simulink model "OCTModelLateralFlight"  (R2018b)
settings: Solver=FixedStepAuto  StartTime=0.0  StopTime=duration_s  FixedStep=0.1  MaxStep=0.1  RelTol=1e-3  AbsTol=1e-3
values from neighbouring files (symbols this model uses):
  constantNormVelBool = 0    [MMadd_ts.m]    (also in controlSurf_ts1.m; lateralFlight_ts.m)
  constantVelBool = 1    [JamesPathFollowingIntegration_ts1.m]    (also in MMadd_ts.m = 0; PathFollowingIntegration_ts1.m; controlSurf_ts1.m = 0; lateralFlight_ts.m = 0)
  constantVelMag = 7    [JamesPathFollowingIntegration_ts1.m]    (also in MMadd_ts.m = 19; PathFollowingIntegration_ts1.m = 10; controlSurf_ts1.m = 19; lateralFlight_ts.m = 34)
  env = ENV.env    [JamesPathFollowingIntegration_ts1.m]    (also in MMadd_ts.m; PathFollowingIntegration_ts1.m; controlSurf_ts1.m; controlSurf_ts2.m)
  kdRollMom = 5*MOI_X    [JamesPathFollowingIntegration_ts1.m]    (also in PathFollowingIntegration_ts1.m; lateralFlight_ts.m)
  kdVelAng = kpVelAng    (= 0.5)    [JamesPathFollowingIntegration_ts1.m]    (also in PathFollowingIntegration_ts1.m = 0.222222222222; lateralFlight_ts.m = 0.222222222222)
  kpRollMom = 2*MOI_X    [JamesPathFollowingIntegration_ts1.m]    (also in PathFollowingIntegration_ts1.m; lateralFlight_ts.m)
  kpVelAng = maxBank/(pi/2)    (= 0.5)    [JamesPathFollowingIntegration_ts1.m]    (also in PathFollowingIntegration_ts1.m = 0.222222222222; lateralFlight_ts.m = 0.222222222222)
  maxBank = 45*pi/180    (= 0.785398163397)    [JamesPathFollowingIntegration_ts1.m]    (also in PathFollowingIntegration_ts1.m = 0.349065850399; lateralFlight_ts.m = 0.349065850399)
  MMAddBool = 0    [JamesPathFollowingIntegration_ts1.m]    (also in MMadd_ts.m = 1; PathFollowingIntegration_ts1.m = 1; controlSurf_ts1.m; controlSurf_ts2.m)
  MMOverrideBool = 1    [JamesPathFollowingIntegration_ts1.m]    (also in MMadd_ts.m = 0; PathFollowingIntegration_ts1.m = 0; controlSurf_ts1.m = 0; lateralFlight_ts.m = 0)
  radialMotionBool = 0    [MMadd_ts.m]    (also in controlSurf_ts1.m; lateralFlight_ts.m)
  startControl = 15    [MMadd_ts.m]    (also in PathFollowingIntegration_ts1.m = 20; controlSurf_ts1.m; controlSurf_ts2.m = 1; controlSurf_ts3.m = 1)
  tauRollMom = .01    (= 0.01)    [JamesPathFollowingIntegration_ts1.m]    (also in PathFollowingIntegration_ts1.m; lateralFlight_ts.m)
  tauVelAng = .01    (= 0.01)    [JamesPathFollowingIntegration_ts1.m]    (also in PathFollowingIntegration_ts1.m; lateralFlight_ts.m)
  vhcl = OCT.vehicle    [JamesPathFollowingIntegration_ts1.m]    (also in MMadd_ts.m; PathFollowingIntegration_ts1.m; controlSurf_ts1.m; controlSurf_ts2.m)
undefined symbols (not defined in the file or in its folder): initAngRates, initializeVariantsFromBlock, Jinv, lateralFlightController, m, Minv, modVehicle000, modVehicle000_cl, plant, plant_cl, sim_param, sixDoFDynamics, sixDoFDynamics_ul, vehicle, vehicle_cl
libraries: vrlib x3, eulAng2RotMat_ul x3, vectorNormalizer_ul x3, setpointToOutput_cl x2, filteredPIDController_ul x2, thrAttachPtKinematics_ul x2, environment_cl x1, cartToSphere_ul x1, schmehlTangentRotation_ul x1, groundStation_cl x1, tethers_cl x1, dragTurbine_ul x1
settings Model: ExtModeTrigDuration=100  Creator=mcobb  LastModifiedBy=James Reed
settings DataIOCC: SaveOutput=off  StateSaveName=tmp_raccel_xout
settings OptimizationCC: EfficientMapNaN2IntZero=off
settings DebuggingCC: SignalRangeChecking=error
settings HardwareCC: TargetBitPerPointer=64  TargetBitPerSizeT=64  TargetBitPerPtrDiffT=64  TargetLongLongMode=on  TargetIntDivRoundTo=Zero  TargetEndianess=LittleEndian  TargetWordSize=64  TargetHWDeviceType=MATLAB Host  ProdEqTarget=off
settings RTWCC: SystemTargetFile=raccel.tlc  TemplateMakefile=raccel_default_tmf  RTWVerbose=off  RTWUseSimCustomCode=on
settings CodeAppCC: GenerateComments=off  MaxIdLength=128  MangleLength=10
settings RaccelTargetCC: GeneratePreprocessorConditionals=Use local settings  MultiInstanceERTCode=off  PreserveStateflowLocalDataDimensions=off  ENABLE_SLEXEC_SSBRIDGE=1  RTWCAPIParams=on

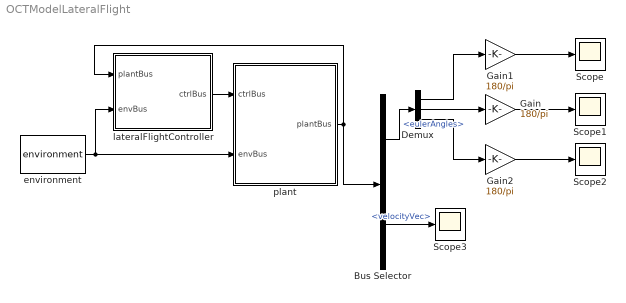
== system OCTModelLateralFlight ==
  Bus Selector : BusSelector  OutputSignals=eulerAngles,velocityVec
  Demux : Demux  Outputs=3
  Gain : Gain  Gain=180/pi
  Gain1 : Gain  Gain=180/pi
  Gain2 : Gain  Gain=180/pi
  Scope{,1..3} (4 alike) : Scope
  environment : environment_cl/environment  SystemSampleTime=-1
  lateralFlightController : Subsystem  AncestorBlock=lateralFlightController/lateralFlightController
  plant : Subsystem  AncestorBlock=plant_cl/plant  VariantControl=VSS_plant_modularPlant
  wires:
  lateralFlightController/1(ctrlBus) -> plant/1(ctrlBus)
  plant/1(plantBus) -> lateralFlightController/1(plantBus), Bus Selector/1
  environment/1 -> lateralFlightController/2(envBus), plant/2(envBus)
  Bus Selector/1 -> Demux/1  "<eulerAngles>"
  Demux/2 -> Gain/1
  Gain/1 -> Scope1/1
  Bus Selector/2 -> Scope3/1  "<velocityVec>"
  Gain2/1 -> Scope2/1
  Gain1/1 -> Scope/1
  Demux/1 -> Gain1/1
  Demux/3 -> Gain2/1

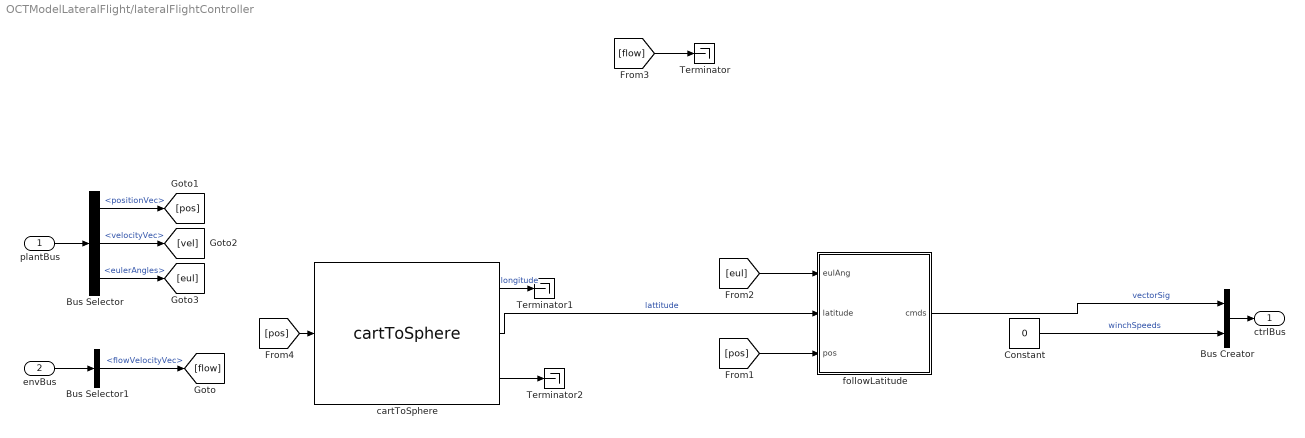
== system OCTModelLateralFlight/lateralFlightController ==
  plantBus : Inport  OutDataTypeStr=Bus: plantBus
  envBus : Inport  Port=2  OutDataTypeStr=Bus: envBus
  Bus Creator : BusCreator  Inputs=2  OutDataTypeStr=Bus: ctrlBus
  Bus Selector : BusSelector  OutputSignals=positionVec,velocityVec,eulerAngles
  Bus Selector1 : BusSelector  OutputSignals=flowVelocityVec
  Constant : Constant  Value=0
  Terminator : Terminator
  Terminator1 : Terminator
  Terminator2 : Terminator
  cartToSphere : cartToSphere_ul/cartToSphere  SystemSampleTime=-1
  followLatitude : Subsystem  mask{kpVelAngMask=kpVelAng, kdVelAngMask=kdVelAng, tauVelAngMask=tauVelAng, kpLMask=kpRollMom, kdLMask=kdRollMom, tauLMask=tauRollMom, maxBankMask=maxBank, latDes=pi/4}
      mask prompts: kpVelAngMask "Proportional Gain Velocity Angle"; kdVelAngMask "Derivative Gain Velocity Angle"; tauVelAngMask "Tau Velocity Angle"; kpLMask "Proportional Gain TanRoll"; kdLMask "Derivative Gain Tanroll"; tauLMask "Tau Roll Moment"; maxBankMask "Max Bank Angle"; latDes "Desired Latitude"
  ctrlBus : Outport  OutDataTypeStr=Bus: ctrlBus
  wires:
  [pos] -> followLatitude/3("pos ")
  cartToSphere/2 -> followLatitude/2("latitude ")  "lattitude"
  cartToSphere/3 -> Terminator2/1
  cartToSphere/1 -> Terminator1/1  "longitude"
  [pos] -> cartToSphere/1
  [flow] -> Terminator/1
  [eul] -> followLatitude/1(eulAng)
  Constant/1 -> Bus Creator/2  "winchSpeeds"
  followLatitude/1(cmds) -> Bus Creator/1  "vectorSig"
  Bus Creator/1 -> ctrlBus/1
  envBus/1 -> Bus Selector1/1
  plantBus/1 -> Bus Selector/1
  Bus Selector/2 -> [vel]  "<velocityVec>"
  Bus Selector1/1 -> [flow]  "<flowVelocityVec>"
  Bus Selector/1 -> [pos]  "<positionVec>"
  Bus Selector/3 -> [eul]  "<eulerAngles>"

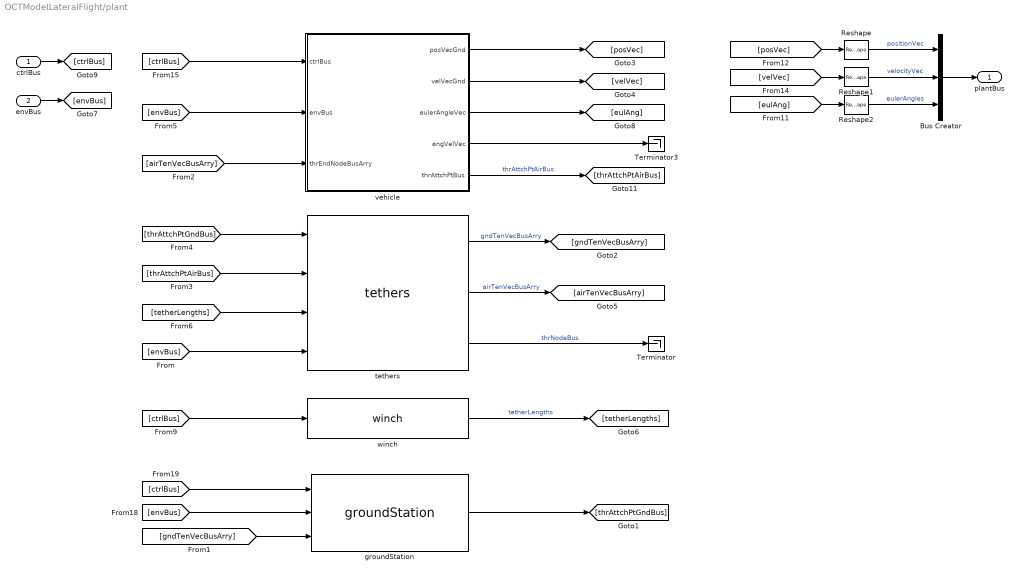
== system OCTModelLateralFlight/plant ==
  ctrlBus : Inport  OutDataTypeStr=Bus: ctrlBus
  envBus : Inport  Port=2  OutDataTypeStr=Bus: envBus
  Bus Creator : BusCreator  Inputs=3  OutDataTypeStr=Bus: plantBus
  Reshape : Reshape  OutputDimensionality=Column vector (2-D)
  Reshape1 : Reshape  OutputDimensionality=Column vector (2-D)
  Reshape2 : Reshape  OutputDimensionality=Column vector (2-D)
  Terminator : Terminator
  Terminator3 : Terminator
  groundStation : groundStation_cl/groundStation  SystemSampleTime=-1
  tethers : tethers_cl/tethers  SystemSampleTime=-1
      link override tether000: numNodes=thr.tether1.numNodes.Value
  vehicle : Subsystem  AncestorBlock=vehicle_cl/vehicle  LoadFcn=initializeVariantsFromBlock(gcb)  InitFcn=initializeVariantsFromBlock(gcb)  StartFcn=initializeVariantsFromBlock(gcb)  Variant=on
      settings: PreSaveFcn=initializeVariantsFromBlock(gcb)
  winch : winch_cl/winch  SystemSampleTime=-1
  plantBus : Outport  OutDataTypeStr=Bus: plantBus
  wires:
  [ctrlBus] -> winch/1
  [envBus] -> vehicle/2(envBus)
  [ctrlBus] -> vehicle/1(ctrlBus)
  [ctrlBus] -> groundStation/1
  [envBus] -> groundStation/2
  [tetherLengths] -> tethers/3
  [thrAttchPtGndBus] -> tethers/1
  [thrAttchPtAirBus] -> tethers/2
  [airTenVecBusArry] -> vehicle/3(thrEndNodeBusArry)
  [gndTenVecBusArry] -> groundStation/3
  tethers/3 -> Terminator/1  "thrNodeBus"
  tethers/2 -> [airTenVecBusArry]  "airTenVecBusArry"
  tethers/1 -> [gndTenVecBusArry]  "gndTenVecBusArry"
  groundStation/1 -> [thrAttchPtGndBus]
  [envBus] -> tethers/4
  vehicle/4(angVelVec) -> Terminator3/1
  vehicle/2(velVecGnd) -> [velVec]
  vehicle/5(thrAttchPtBus) -> [thrAttchPtAirBus]  "thrAttchPtAirBus"
  vehicle/1(posVecGnd) -> [posVec]
  vehicle/3(eulerAngleVec) -> [eulAng]
  [eulAng] -> Reshape2/1
  [velVec] -> Reshape1/1
  [posVec] -> Reshape/1
  winch/1 -> [tetherLengths]  "tetherLengths"
  Reshape1/1 -> Bus Creator/2  "velocityVec"
  Reshape2/1 -> Bus Creator/3  "eulerAngles"
  Reshape/1 -> Bus Creator/1  "positionVec"
  Bus Creator/1 -> plantBus/1
  ctrlBus/1 -> [ctrlBus]
  envBus/1 -> [envBus]

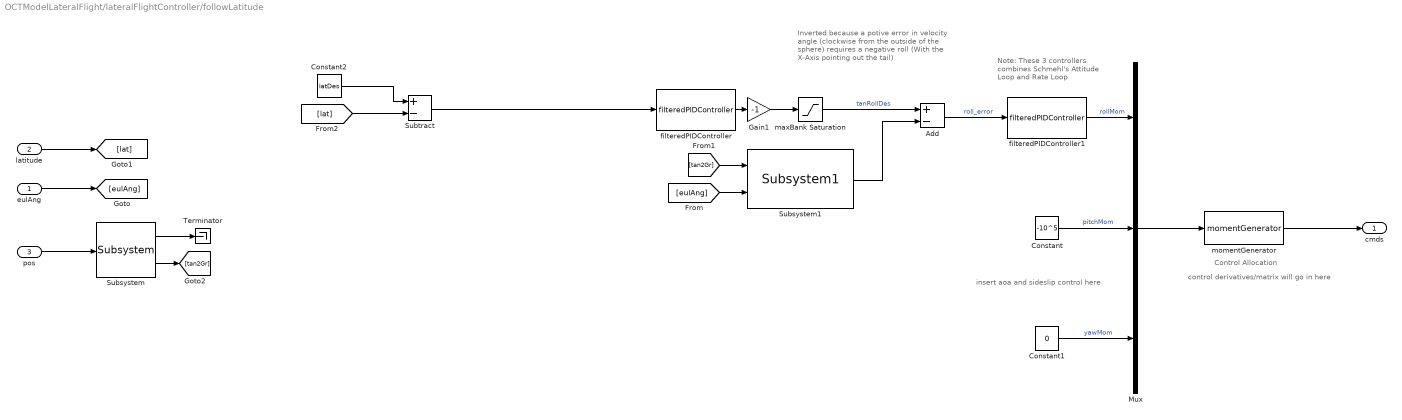
== system OCTModelLateralFlight/lateralFlightController/followLatitude ==
  note: Note: These 3 controllers
      | combines Schmehl's Attitude
      | Loop and Rate Loop
  note: Inverted because a potive error
      | in velocity angle (clockwise from the
      | outside of the sphere) requires a negative
      | roll (With the X-Axis pointing out the tail)
  note: Control Allocation
  note: insert aoa and sideslip control here
  note: control derivatives/matrix will go in here
  eulAng : Inport
  "latitude " : Inport  Port=2
  "pos " : Inport  Port=3
  Add : Sum  Inputs=+-
  Constant : Constant  Value=-10^5
  Constant1 : Constant  Value=0
  Constant2 : Constant  Value=latDes
  Gain1 : Gain  Gain=-1
  Mux : Mux  Inputs=3
  Subsystem : schmehlTangentRotation_ul/Subsystem  SystemSampleTime=-1
  Subsystem1 : setpointToOutput_cl/Subsystem/Subsystem1  SystemSampleTime=-1
  Subtract : Sum  Inputs=+-
  Terminator : Terminator
  filteredPIDController : filteredPIDController_ul/filteredPIDController  kp=kpVelAngMask  ki=0  kd=kdVelAngMask  Value=tauVelAngMask
  filteredPIDController1 : filteredPIDController_ul/filteredPIDController  kp=kpLMask  ki=0  kd=kdLMask  Value=tauLMask
  maxBank Saturation : Saturate  UpperLimit=maxBankMask  LowerLimit=-maxBankMask
  momentGenerator : setpointToOutput_cl/Subsystem/momentGenerator  SystemSampleTime=-1
  cmds : Outport
  wires:
  Subsystem/1 -> Terminator/1
  Subsystem/2 -> [tan2Gr]
  "pos "/1 -> Subsystem/1
  Subtract/1 -> filteredPIDController/1
  Constant2/1 -> Subtract/1
  [lat] -> Subtract/2
  "latitude "/1 -> [lat]
  momentGenerator/1 -> cmds/1
  Mux/1 -> momentGenerator/1
  maxBank Saturation/1 -> Add/1  "tanRollDes"
  Constant/1 -> Mux/2  "pitchMom"
  [eulAng] -> Subsystem1/2
  filteredPIDController1/1 -> Mux/1  "rollMom"
  filteredPIDController/1 -> Gain1/1
  eulAng/1 -> [eulAng]
  Subsystem1/1 -> Add/2
  Gain1/1 -> maxBank Saturation/1
  Add/1 -> filteredPIDController1/1  "roll_error"
  Constant1/1 -> Mux/3  "yawMom"
  [tan2Gr] -> Subsystem1/1

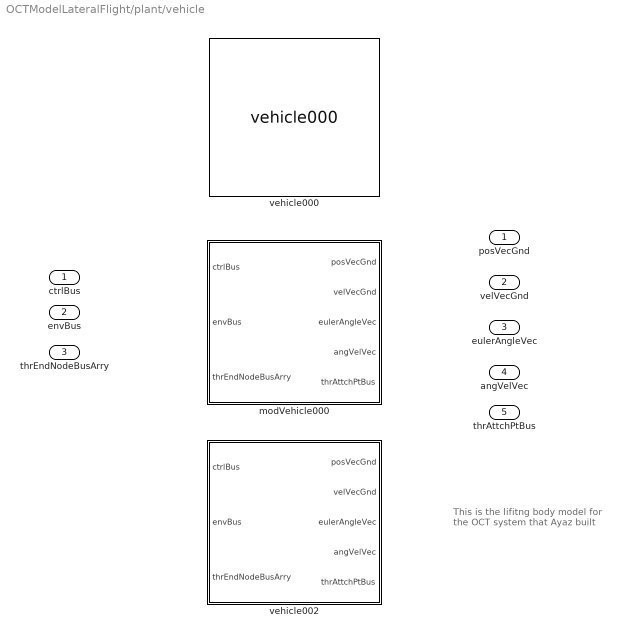
== system OCTModelLateralFlight/plant/vehicle ==
  note: This is the lifitng body model for the OCT system that Ayaz built
  ctrlBus : Inport  OutDataTypeStr=Bus: ctrlBus
  envBus : Inport  Port=2  OutDataTypeStr=Bus: envBus
  thrEndNodeBusArry : Inport  Port=3
  modVehicle000 : Subsystem  AncestorBlock=modVehicle000_cl/modVehicle000  VariantControl=VSS_vehicle_modVehicle000  mask{vcl=vhcl, rho=env.water.density.Value, grav=env.gravAccel.Value}
      mask prompts: vcl "Vehicle"; rho "Fluid Density"; grav "Gravity"
      mask DialogControl Container9 Prompt: General
      mask DialogControl Container5 Prompt: Vehicle object
      mask DialogControl ParameterGroupVar Prompt: Environmental
      mask Display:
      | image('kite.jpg',[100 100 601 528]/4,'on')
      | 
      | port_label('input',1,'ctrlBus')
      | port_label('input',2,'envBus')
      | port_label('input',3,'thrEndNodeBusArry')
      | 
      | port_label('output',1,'posVecGnd')
      | port_label('output',2,'velVecGnd')
      | port_label('output',3,'eulAng')
      | port_label('output',4,'angVelVec')
      | port_label('output',5,'thrAttchPtBus')
  vehicle000 : vehicle000_cl/vehicle000  VariantControl=VSS_vehicle_vehicle000  vcl=vhcl  rho=env.water.density.Value  grav=env.gravAccel.Value
  vehicle002 : Subsystem  VariantControl=VSS_vehicle_vehicle002
      mask init:
      | load('OrginalOCctModelVars');
  posVecGnd : Outport
  velVecGnd : Outport  Port=2
  eulerAngleVec : Outport  Port=3
  angVelVec : Outport  Port=4
  thrAttchPtBus : Outport  Port=5

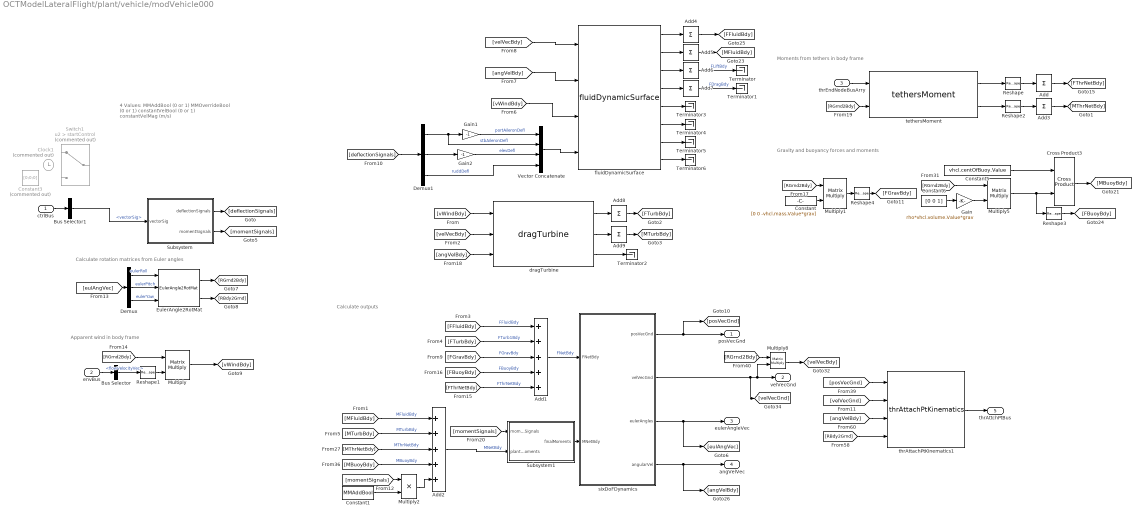
== system OCTModelLateralFlight/plant/vehicle/modVehicle000 ==
  note: Moments from tethers in body frame
  note: Gravity and buoyancy forces and moments
  note: Calculate rotation matrices from Euler angles
  note: Apparent wind in body frame
  note: Calculate outputs
  note: 4 Values:
      | MMAddBool (0 or 1)
      | MMOverrideBool (0 or 1)
      | constantVelBool (0 or 1)
      | constantVelMag (m/s)
  ctrlBus : Inport  OutDataTypeStr=Bus: ctrlBus
  envBus : Inport  Port=2  OutDataTypeStr=Bus: envBus
  thrEndNodeBusArry : Inport  Port=3
  Add : Sum  Inputs=+  CollapseMode=Specified dimension  CollapseDim=2
  Add1 : Sum  Inputs=+++++
  Add2 : Sum  Inputs=+++++
  Add3 : Sum  Inputs=+  CollapseMode=Specified dimension  CollapseDim=2
  Add{4..9} (6 alike) : Sum  Inputs=1  CollapseMode=Specified dimension  CollapseDim=2
  Bus Selector : BusSelector  OutputSignals=flowVelocityVec
  Bus Selector1 : BusSelector  OutputSignals=vectorSig
  Clock1 : Clock  Commented=on
  Constant : Constant  Value=[0 0 -vhcl.mass.Value*grav]
  Constant1 : Constant  Value=MMAddBool
  Constant3 : Constant  Commented=on  Value=[0;0;0]
  Constant5 : Constant  Value=vhcl.centOfBuoy.Value
  Constant6 : Constant  Value=[0 0 1]
  Cross Product3 : vrlib/Utilities/Cross Product
      settings: SourceProductBaseCode=VR
  Demux : Demux  Outputs=3
  Demux1 : Demux  Outputs=3
  EulerAngle2RotMat : eulAng2RotMat_ul/EulerAngle2RotMat  SystemSampleTime=-1
  Gain : Gain  Gain=rho*vhcl.volume.Value*grav
  Gain1 : Gain  Gain=-1
  Gain2 : Gain  Gain=-1
  Multiply{,1,5,8} (4 alike) : Product  Multiplication=Matrix(*)
  Multiply2 : Product
  Reshape : Reshape  OutputDimensionality=Customize  OutputDimensions=[3 vhcl.numTethers.Value]
  Reshape1 : Reshape  OutputDimensionality=Column vector (2-D)
  Reshape2 : Reshape  OutputDimensionality=Customize  OutputDimensions=[3 vhcl.numTethers.Value]
  Reshape3 : Reshape  OutputDimensionality=Column vector (2-D)
  Reshape4 : Reshape  OutputDimensionality=Column vector (2-D)
  Subsystem : Subsystem
  Subsystem1 : Subsystem
  Switch1 : Switch  Commented=on  Criteria=u2 > Threshold  Threshold=startControl
  Terminator{,1..6} (7 alike) : Terminator
  Vector Concatenate : Concatenate  NumInputs=4
  dragTurbine : dragTurbine_ul/dragTurbine  rho_fluid=rho  turb_struct=vhcl.struct('OCT.turb')
  fluidDynamicSurface : fluidDynamicSurface_cl/fluidDynamicSurface  aeroStruct=vcl.struct('OCT.aeroSurf')  fluidDensity=rho
  sixDoFDynamics : Subsystem  AncestorBlock=sixDoFDynamics_ul/sixDoFDynamics  mask{M=vhcl.mass.Value, J=vhcl.inertia.Value, initPos=vhcl.initPosVecGnd.Value, initVel=vhcl.initVelVecGnd.Value, initEulAngs=vhcl.initEulAngBdy.Value, initAngVel=vhcl.initAngVelVecBdy.Value}
      mask prompts: M "Mass"; J "Inertia matrix"; initPos "Initial position"; initVel "Initial velocity"; initEulAngs "Initial Euler Angles"; initAngVel "Initial Angular Velocity Vec"
      mask init:
      | sixDoFDynamics_init
  tethersMoment : tethersMoment_cl/tethersMoment  arms=vhcl.struct('OCT.thrAttch')
  thrAttachPtKinematics1 : thrAttachPtKinematics_ul/thrAttachPtKinematics  atchPts=vhcl.struct('OCT.thrAttch')
  posVecGnd : Outport
  velVecGnd : Outport  Port=2
  eulerAngleVec : Outport  Port=3
  angVelVec : Outport  Port=4
  thrAttchPtBus : Outport  Port=5
  wires:
  Bus Selector1/1 -> Subsystem/1(vectorSig)  "<vectorSig>"
  fluidDynamicSurface/8 -> Terminator6/1
  Subsystem/2(momentSignals) -> [momentSignals]
  Reshape4/1 -> [FGravBdy]
  Multiply1/1 -> Reshape4/1
  Reshape3/1 -> [FBuoyBdy]
  fluidDynamicSurface/6 -> Terminator4/1
  fluidDynamicSurface/7 -> Terminator5/1
  fluidDynamicSurface/5 -> Terminator3/1
  Constant1/1 -> Multiply2/2
  Multiply2/1 -> Add2/5
  [momentSignals] -> Multiply2/1
  sixDoFDynamics/2(velVecGnd) -> [velVecGnd], Multiply8/2, velVecGnd/1
  [momentSignals] -> Subsystem1/1(momentSignals)
  Add2/1 -> Subsystem1/2("plantCreatedMoments ")  "MNetBdy"
  Subsystem1/1(finalMoments) -> sixDoFDynamics/2(MNetBdy)
  Subsystem/1(deflectionSignals) -> [deflectionSignals]
  Gain2/1 -> Vector Concatenate/3  "elevDefl"
  Demux1/1 -> Gain1/1, Vector Concatenate/2  "stbAileronDefl"
  Gain1/1 -> Vector Concatenate/1  "portAileronDefl"
  Demux1/2 -> Gain2/1
  Demux1/3 -> Vector Concatenate/4  "ruddDefl"
  [deflectionSignals] -> Demux1/1
  ctrlBus/1 -> Bus Selector1/1
  Vector Concatenate/1 -> fluidDynamicSurface/4
  Gain/1 -> Multiply5/2
  [FGravBdy] -> Add1/3  "FGravBdy"
  [FBuoyBdy] -> Add1/4  "FBuoyBdy"
  [FThrNetBdy] -> Add1/5  "FThrNetBdy"
  [MBuoyBdy] -> Add2/4  "MBuoyBdy"
  [angVelBdy] -> dragTurbine/3
  [velVecBdy] -> dragTurbine/2
  [vWindBdy] -> dragTurbine/1
  dragTurbine/3 -> Terminator2/1
  Add9/1 -> [MTurbBdy]
  Add8/1 -> [FTurbBdy]
  dragTurbine/2 -> Add9/1
  dragTurbine/1 -> Add8/1
  Add7/1 -> Terminator1/1  "FDragBdy"
  Add6/1 -> Terminator/1  "FLiftBdy"
  Add5/1 -> [MFluidBdy]
  Add4/1 -> [FFluidBdy]
  [velVecBdy] -> fluidDynamicSurface/1
  [angVelBdy] -> fluidDynamicSurface/2
  [vWindBdy] -> fluidDynamicSurface/3
  fluidDynamicSurface/4 -> Add7/1
  fluidDynamicSurface/3 -> Add6/1
  fluidDynamicSurface/1 -> Add4/1
  envBus/1 -> Bus Selector/1
  Add1/1 -> sixDoFDynamics/1(FNetBdy)  "FNetBdy"
  tethersMoment/2 -> Reshape2/1
  Reshape2/1 -> Add3/1
  Add3/1 -> [MThrNetBdy]
  Reshape1/1 -> Multiply/2
  [RGrnd2Bdy] -> tethersMoment/2
  Add/1 -> [FThrNetBdy]
  Reshape/1 -> Add/1
  tethersMoment/1 -> Reshape/1
  [velVecGnd] -> thrAttachPtKinematics1/2
  [RBdy2Grnd] -> thrAttachPtKinematics1/4
  [posVecGnd] -> thrAttachPtKinematics1/1
  thrAttachPtKinematics1/1 -> thrAttchPtBus/1
  [angVelBdy] -> thrAttachPtKinematics1/3
  [RGrnd2Bdy] -> Multiply8/1
  Multiply8/1 -> [velVecBdy]
  sixDoFDynamics/1(posVecGnd) -> posVecGnd/1, [posVecGnd]
  fluidDynamicSurface/2 -> Add5/1
  Constant/1 -> Multiply1/2
  [FTurbBdy] -> Add1/2  "FTurb1Bdy"
  [FFluidBdy] -> Add1/1  "FFluidBdy"
  sixDoFDynamics/4(angularVel) -> angVelVec/1, [angVelBdy]
  sixDoFDynamics/3(eulerAngles) -> eulerAngleVec/1, [eulAngVec]
  [MTurbBdy] -> Add2/2  "MTurbBdy"
  [MThrNetBdy] -> Add2/3  "MThrNetBdy"
  [MFluidBdy] -> Add2/1  "MFluidBdy"
  Constant5/1 -> Cross Product3/1
  Cross Product3/1 -> [MBuoyBdy]
  [RGrnd2Bdy] -> Multiply5/1
  Multiply5/1 -> Reshape3/1, Cross Product3/2
  Constant6/1 -> Gain/1
  thrEndNodeBusArry/1 -> tethersMoment/1
  [RGrnd2Bdy] -> Multiply1/1
  Multiply/1 -> [vWindBdy]
  [RGrnd2Bdy] -> Multiply/1
  EulerAngle2RotMat/2 -> [RBdy2Grnd]
  EulerAngle2RotMat/1 -> [RGrnd2Bdy]
  Demux/3 -> EulerAngle2RotMat/3  "eulerYaw"
  Demux/1 -> EulerAngle2RotMat/1  "eulerRoll"
  Demux/2 -> EulerAngle2RotMat/2  "eulerPitch"
  [eulAngVec] -> Demux/1
  Bus Selector/1 -> Reshape1/1  "<flowVelocityVec>"

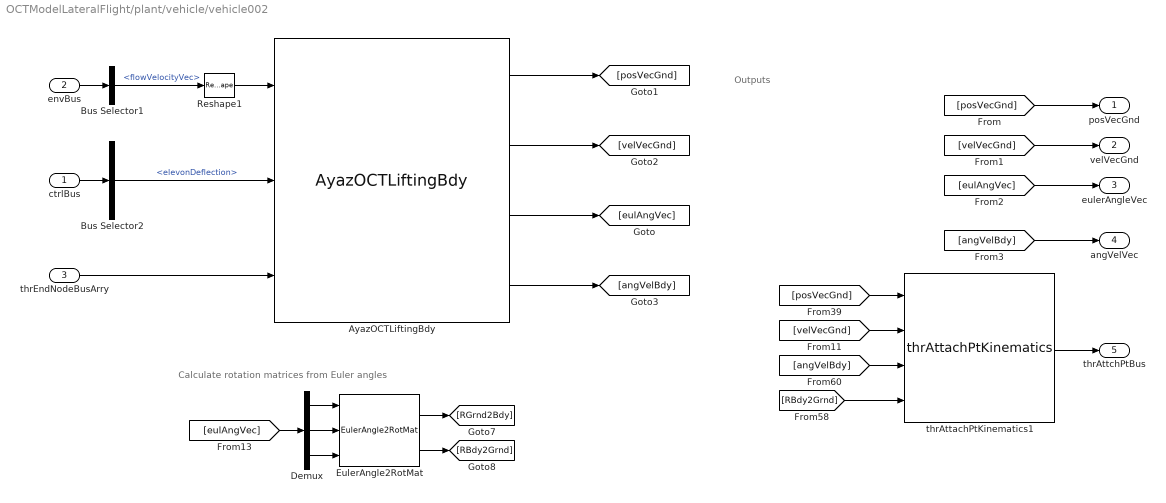
== system OCTModelLateralFlight/plant/vehicle/vehicle002 ==
  note: Calculate rotation matrices from Euler angles
  note: Outputs
  ctrlBus : Inport  OutDataTypeStr=Bus: ctrlBus
  envBus : Inport  Port=2  OutDataTypeStr=Bus: envBus
  thrEndNodeBusArry : Inport  Port=3
  AyazOCTLiftingBdy : AyazOctLiftingBdy_cl/AyazOCTLiftingBdy  sim_param=sim_param  initCon=origOCT_iniCon
  Bus Selector1 : BusSelector  OutputSignals=flowVelocityVec
  Bus Selector2 : BusSelector  OutputSignals=elevonDeflection
  Demux : Demux  Outputs=3
  EulerAngle2RotMat : eulAng2RotMat_ul/EulerAngle2RotMat  SystemSampleTime=-1
  Reshape1 : Reshape  OutputDimensionality=Column vector (2-D)
  thrAttachPtKinematics1 : thrAttachPtKinematics_ul/thrAttachPtKinematics  atchPts=[sim_param.tether_imp_nodes.R1n_cm,sim_param.tether_imp_nodes.R2n_cm,sim_param.tether_imp_nodes.R3n_cm]
  posVecGnd : Outport
  velVecGnd : Outport  Port=2
  eulerAngleVec : Outport  Port=3
  angVelVec : Outport  Port=4
  thrAttchPtBus : Outport  Port=5
  wires:
  [angVelBdy] -> angVelVec/1
  [eulAngVec] -> eulerAngleVec/1
  [velVecGnd] -> velVecGnd/1
  [posVecGnd] -> posVecGnd/1
  AyazOCTLiftingBdy/4 -> [angVelBdy]
  AyazOCTLiftingBdy/2 -> [velVecGnd]
  AyazOCTLiftingBdy/1 -> [posVecGnd]
  AyazOCTLiftingBdy/3 -> [eulAngVec]
  EulerAngle2RotMat/2 -> [RBdy2Grnd]
  EulerAngle2RotMat/1 -> [RGrnd2Bdy]
  Demux/1 -> EulerAngle2RotMat/1
  Demux/2 -> EulerAngle2RotMat/2
  [eulAngVec] -> Demux/1
  Demux/3 -> EulerAngle2RotMat/3
  [velVecGnd] -> thrAttachPtKinematics1/2
  [angVelBdy] -> thrAttachPtKinematics1/3
  thrAttachPtKinematics1/1 -> thrAttchPtBus/1
  [RBdy2Grnd] -> thrAttachPtKinematics1/4
  [posVecGnd] -> thrAttachPtKinematics1/1
  thrEndNodeBusArry/1 -> AyazOCTLiftingBdy/3
  Bus Selector2/1 -> AyazOCTLiftingBdy/2  "<elevonDeflection>"
  ctrlBus/1 -> Bus Selector2/1
  envBus/1 -> Bus Selector1/1
  Reshape1/1 -> AyazOCTLiftingBdy/1
  Bus Selector1/1 -> Reshape1/1  "<flowVelocityVec>"

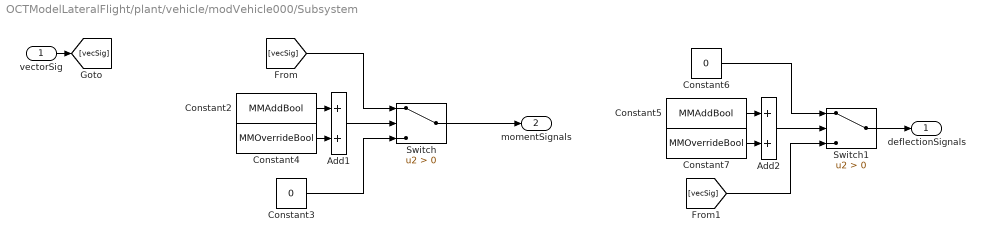
== system OCTModelLateralFlight/plant/vehicle/modVehicle000/Subsystem ==
  vectorSig : Inport
  Add1 : Sum
  Add2 : Sum
  Constant2 : Constant  Value=MMAddBool
  Constant3 : Constant  Value=0
  Constant4 : Constant  Value=MMOverrideBool
  Constant5 : Constant  Value=MMAddBool
  Constant6 : Constant  Value=0
  Constant7 : Constant  Value=MMOverrideBool
  Switch : Switch  Criteria=u2 > Threshold
  Switch1 : Switch  Criteria=u2 > Threshold
  deflectionSignals : Outport
  momentSignals : Outport  Port=2
  wires:
  Constant6/1 -> Switch1/1
  vectorSig/1 -> [vecSig]
  Switch1/1 -> deflectionSignals/1
  Add2/1 -> Switch1/2
  Constant5/1 -> Add2/1
  Constant7/1 -> Add2/2
  [vecSig] -> Switch1/3
  Switch/1 -> momentSignals/1
  Constant4/1 -> Add1/2
  Constant2/1 -> Add1/1
  Add1/1 -> Switch/2
  [vecSig] -> Switch/1
  Constant3/1 -> Switch/3

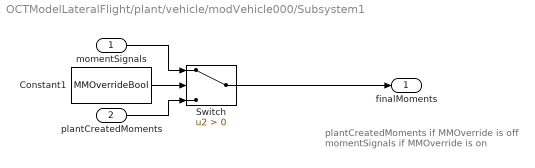
== system OCTModelLateralFlight/plant/vehicle/modVehicle000/Subsystem1 ==
  note: plantCreatedMoments if MMOverride is off
      | momentSignals if MMOverride is on
  momentSignals : Inport
  "plantCreatedMoments " : Inport  Port=2
  Constant1 : Constant  Value=MMOverrideBool
  Switch : Switch  Criteria=u2 > Threshold
  finalMoments : Outport
  wires:
  Switch/1 -> finalMoments/1
  "plantCreatedMoments "/1 -> Switch/3
  momentSignals/1 -> Switch/1
  Constant1/1 -> Switch/2

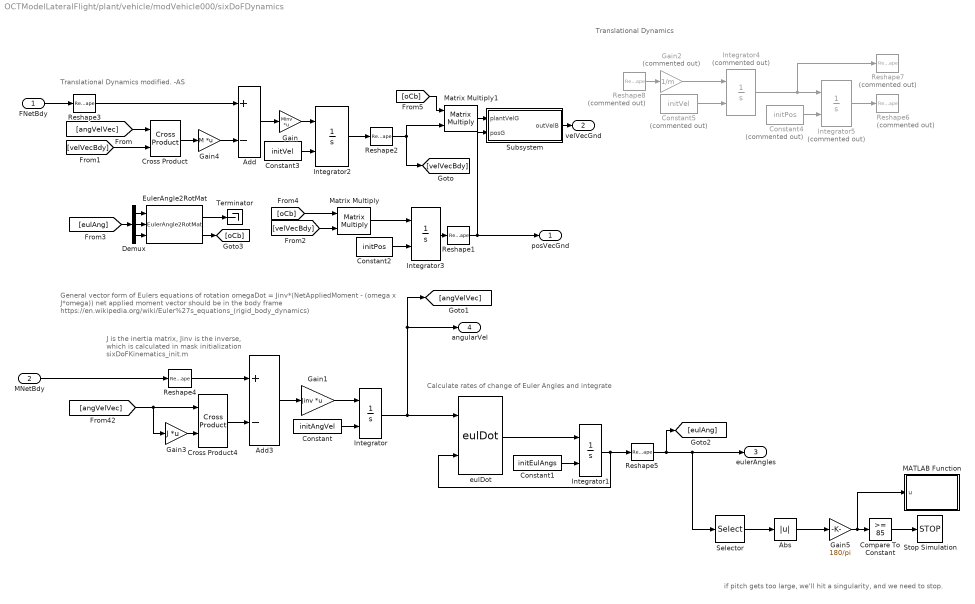
== system OCTModelLateralFlight/plant/vehicle/modVehicle000/sixDoFDynamics ==
  note: if pitch gets too large, we'll hit a singularity, and we need to stop.
  note: Translational Dynamics modified. -AS
  note: Calculate rates of change of Euler Angles and integrate
  note: General vector form of Eulers equations of rotation
      | omegaDot = Jinv*(NetAppliedMoment - (omega x J*omega))
      | net applied moment vector should be in the body frame
      | https://en.wikipedia.org/wiki/Euler%27s_equations_(rigid_body_dynamics)
  note: J is the inertia matrix, Jinv is the inverse,
      | which is calculated in mask initialization
      | sixDoFKinematics_init.m
  note: Translational Dynamics
  FNetBdy : Inport
  MNetBdy : Inport  Port=2
  Abs : Abs
  Add : Sum  Inputs=+-
  Add3 : Sum  Inputs=+-
  Compare To Constant : simulink/Logic and Bit Operations/Compare To Constant  relop=>=  const=85  OutDataTypeStr=boolean
  Constant : Constant  Value=initAngVel
  Constant1 : Constant  Value=initEulAngs
  Constant2 : Constant  Value=initPos
  Constant3 : Constant  Value=initVel
  Constant4 : Constant  Commented=on  Value=initPos
  Constant5 : Constant  Commented=on  Value=initVel
  Cross Product : vrlib/Utilities/Cross Product
      settings: SourceProductBaseCode=VR
  Cross Product4 : vrlib/Utilities/Cross Product
      settings: SourceProductBaseCode=VR
  Demux : Demux  Outputs=3
  EulerAngle2RotMat : eulAng2RotMat_ul/EulerAngle2RotMat  SystemSampleTime=-1
  Gain : Gain  Gain=Minv  Multiplication=Matrix(K*u)
  Gain1 : Gain  Gain=Jinv  Multiplication=Matrix(K*u)
  Gain2 : Gain  Commented=on  Gain=1/m
  Gain3 : Gain  Gain=J  Multiplication=Matrix(K*u)
  Gain4 : Gain  Gain=M  Multiplication=Matrix(K*u)
  Gain5 : Gain  Gain=180/pi
  Integrator : Integrator  InitialConditionSource=external  InitialCondition=initAngRates
  Integrator1 : Integrator  InitialConditionSource=external  InitialCondition=initEulAngs
  Integrator2 : Integrator  InitialConditionSource=external  InitialCondition=initVel
  Integrator3 : Integrator  InitialConditionSource=external  InitialCondition=initPos
  Integrator4 : Integrator  Commented=on  InitialConditionSource=external  InitialCondition=initVel
  Integrator5 : Integrator  Commented=on  InitialConditionSource=external  InitialCondition=initPos
  MATLAB Function : MATLAB Function  TreatAsAtomicUnit=on
  Matrix Multiply : Product  Multiplication=Matrix(*)
  Matrix Multiply1 : Product  Multiplication=Matrix(*)
  Reshape{1..5} (5 alike) : Reshape  OutputDimensionality=Column vector (2-D)
  Reshape6 : Reshape  Commented=on  OutputDimensionality=Column vector (2-D)
  Reshape7 : Reshape  Commented=on  OutputDimensionality=Column vector (2-D)
  Reshape8 : Reshape  Commented=on  OutputDimensionality=Column vector (2-D)
  Selector : Selector  InputPortWidth=3  IndexOptions=Index vector (dialog)  Indices=2  OutputSizes=1
  Stop Simulation : Stop
  Subsystem : Subsystem
  Terminator : Terminator
  eulDot : eulDot/eulDot  SystemSampleTime=-1
  posVecGnd : Outport
  velVecGnd : Outport  Port=2
  eulerAngles : Outport  Port=3
  angularVel : Outport  Port=4
  wires:
  Subsystem/1("outVelB ") -> velVecGnd/1
  Matrix Multiply1/1 -> Subsystem/1(plantVelG)
  Compare To Constant/1 -> Stop Simulation/1
  Reshape2/1 -> Matrix Multiply1/2, [velVecBdy]
  MNetBdy/1 -> Reshape4/1
  [angVelVec] -> Cross Product4/1, Gain3/1
  Gain3/1 -> Cross Product4/2
  Integrator/1 -> eulDot/1, angularVel/1, [angVelVec]
  Add3/1 -> Gain1/1
  Integrator1/1 -> eulDot/2, Reshape5/1
  Gain1/1 -> Integrator/1
  Cross Product4/1 -> Add3/2
  FNetBdy/1 -> Reshape3/1
  Integrator3/1 -> Reshape1/1
  Constant/1 -> Integrator/2
  eulDot/1 -> Integrator1/1
  Constant1/1 -> Integrator1/2
  Constant2/1 -> Integrator3/2
  Constant3/1 -> Integrator2/2
  Reshape4/1 -> Add3/1
  Reshape5/1 -> [eulAng], Selector/1, eulerAngles/1
  Constant4/1 -> Integrator5/2
  Integrator5/1 -> Reshape6/1
  Constant5/1 -> Integrator4/2
  Integrator4/1 -> Reshape7/1, Integrator5/1
  Gain2/1 -> Integrator4/1
  Reshape8/1 -> Gain2/1
  Cross Product/1 -> Gain4/1
  Reshape3/1 -> Add/1
  Gain4/1 -> Add/2
  Add/1 -> Gain/1
  Gain/1 -> Integrator2/1
  [angVelVec] -> Cross Product/1
  [velVecBdy] -> Cross Product/2
  Integrator2/1 -> Reshape2/1
  [eulAng] -> Demux/1
  Demux/1 -> EulerAngle2RotMat/1
  Demux/2 -> EulerAngle2RotMat/2
  Demux/3 -> EulerAngle2RotMat/3
  [velVecBdy] -> Matrix Multiply/2
  Matrix Multiply/1 -> Integrator3/1
  Reshape1/1 -> Subsystem/2(posG), posVecGnd/1
  EulerAngle2RotMat/1 -> Terminator/1
  EulerAngle2RotMat/2 -> [oCb]
  [oCb] -> Matrix Multiply/1
  [oCb] -> Matrix Multiply1/1
  Selector/1 -> Abs/1
  Abs/1 -> Gain5/1
  Gain5/1 -> Compare To Constant/1, MATLAB Function/1(u)

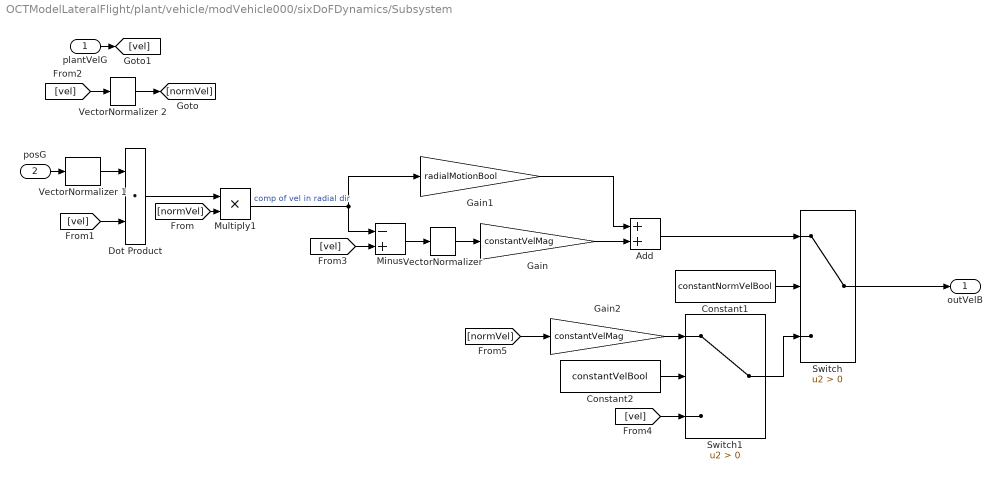
== system OCTModelLateralFlight/plant/vehicle/modVehicle000/sixDoFDynamics/Subsystem ==
  plantVelG : Inport
  posG : Inport  Port=2
  Add : Sum
  Constant1 : Constant  Value=constantNormVelBool  VectorParams1D=off
  Constant2 : Constant  Value=constantVelBool  VectorParams1D=off
  Dot Product : DotProduct  InputSameDT=on  OutDataTypeStr=Inherit: Inherit via internal rule
  Gain : Gain  Gain=constantVelMag
  Gain1 : Gain  Gain=radialMotionBool
  Gain2 : Gain  Gain=constantVelMag
  Minus : Sum  Inputs=-+
  Multiply1 : Product
  Switch : Switch  Criteria=u2 > Threshold
  Switch1 : Switch  Criteria=u2 > Threshold
  "VectorNormalizer " : vectorNormalizer_ul/VectorNormalizer   SystemSampleTime=-1
  VectorNormalizer 1 : vectorNormalizer_ul/VectorNormalizer   SystemSampleTime=-1
  VectorNormalizer 2 : vectorNormalizer_ul/VectorNormalizer   SystemSampleTime=-1
  "outVelB " : Outport
  wires:
  Gain2/1 -> Switch1/1
  [normVel] -> Gain2/1
  Constant2/1 -> Switch1/2
  [vel] -> Switch1/3
  Switch1/1 -> Switch/3
  [vel] -> Minus/2
  [vel] -> VectorNormalizer 2/1
  [vel] -> Dot Product/2
  plantVelG/1 -> [vel]
  [normVel] -> Multiply1/2
  Dot Product/1 -> Multiply1/1
  VectorNormalizer 2/1 -> [normVel]
  Gain1/1 -> Add/1
  Multiply1/1 -> Gain1/1, Minus/1  "comp of vel in radial dir"
  Gain/1 -> Add/2
  Minus/1 -> "VectorNormalizer "/1
  VectorNormalizer 1/1 -> Dot Product/1
  posG/1 -> VectorNormalizer 1/1
  "VectorNormalizer "/1 -> Gain/1
  Constant1/1 -> Switch/2
  Switch/1 -> "outVelB "/1
  Add/1 -> Switch/1

== matlab function OCTModelLateralFlight/plant/vehicle/modVehicle000/sixDoFDynamics/MATLAB Function ==
  data: u input
function fcn(u)
    if u>85
        fprintf("Executed Stop because pitch = %4.2f\n",u)
    end
end
